simulink model "IMU_INS_Data"  (R2023b)
settings: Solver=VariableStepAuto  StartTime=0.0  StopTime=4  RelTol=1e-3
undefined symbols (not defined in the file): DiscIntNeverNeededParam, fractalcoef
libraries: simulink x3, sim3dautolib x2, mspsensorlib x1, sensorinslib x1, sim3dlib x1
settings Model: Creator=Hazem Abdelaziz  LastModifiedBy=Hazem Abdelaziz

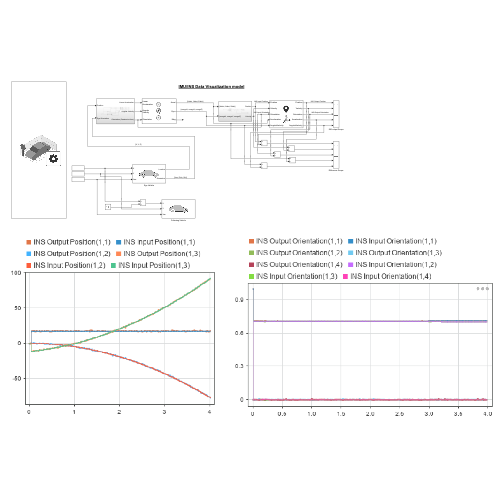
[thumbnail: Simulink's stored preview of the top-level diagram]
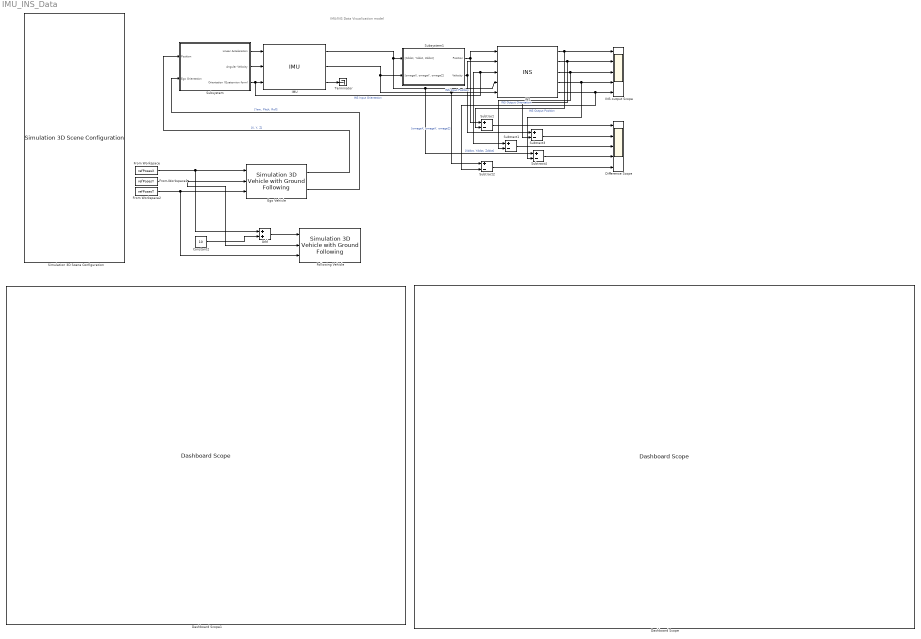
== system IMU_INS_Data ==
  note: IMU/INS Data Visualization model
  Add : Sum
  Constant2 : Constant  Value=10
  Dashboard Scope : DashboardScope  NormalizeYAxis=on
  Dashboard Scope1 : DashboardScope  NormalizeYAxis=on
  Difference Scope : Scope  NumInputPorts=5
  Ego Vehicle : sim3dautolib/Simulation 3D Vehicle with Ground Following  Priority=-1  PassVehMesh=Sedan  MeshPath=/MathWorksAutomotiveContent/Vehicles/Muscle/Meshes/SK_MuscleCar.SK_MuscleCar  TrackWidth=1.9  WheelBase=3  WheelRadius=0.35  VehColor=Black  InitialPos=[0, 0, 0]  InitialRot=[0, 0, 0]  ActorName=SimulinkVehicle1  SampleTime=-1  ActorType=SimulinkVehicle  ID=1  aMode=3  ActorTag=SimulinkVehicle1  CoordinateScheme=ISO  VehLightsControl=off  HeadlightColor=[ 1, 1, 1 ]  HighBeamIntensity=100000  LowBeamIntensity=60000  HighBeamConeAngle=70  LowBeamConeAngle=70  LeftHeadlightOrientation=[ 0, 0 ]  RightHeadlightOrientation=[ 0, 0 ]  BrakelightIntensity=500  ReverselightIntensity=500  SignallightIntensity=500  SignallightPeriod=1  SignalPulseWidth=50  TransformOutportEnabled=on
      settings: LibrarySourceBlock=drivingsim3d/Simulation 3D Vehicle with Ground Following
  Following Vehicle : sim3dautolib/Simulation 3D Vehicle with Ground Following  Priority=-1  PassVehMesh=Sedan  MeshPath=/MathWorksAutomotiveContent/Vehicles/Muscle/Meshes/SK_MuscleCar.SK_MuscleCar  TrackWidth=1.9  WheelBase=3  WheelRadius=0.35  VehColor=Red  InitialPos=[0, 0, 0]  InitialRot=[0, 0, 0]  ActorName=SimulinkVehicle2  SampleTime=-1  ActorType=SimulinkVehicle  ID=2  aMode=3  ActorTag=SimulinkVehicle2  CoordinateScheme=ISO  VehLightsControl=off  HeadlightColor=[ 1, 1, 1 ]  HighBeamIntensity=100000  LowBeamIntensity=60000  HighBeamConeAngle=70  LowBeamConeAngle=70  LeftHeadlightOrientation=[ 0, 0 ]  RightHeadlightOrientation=[ 0, 0 ]  BrakelightIntensity=500  ReverselightIntensity=500  SignallightIntensity=500  SignallightPeriod=1  SignalPulseWidth=50  TransformOutportEnabled=off
      settings: LibrarySourceBlock=drivingsim3d/Simulation 3D Vehicle with Ground Following
  From Workspace : FromWorkspace  VariableName=refPosesX  OutputAfterFinalValue=Holding final value
  From Workspace1 : FromWorkspace  VariableName=refPosesY  OutputAfterFinalValue=Holding final value
  From Workspace2 : FromWorkspace  VariableName=refPosesT  Interpolate=off  OutputAfterFinalValue=Holding final value
  IMU : mspsensorlib/IMU  DispRefFrame=ENU  TemperaturePort=off  Temperature=25  MagneticFieldPort=off  MagneticFieldNED=[ 27.5550, -2.4169, -16.0849 ]  MagneticFieldENU=[-2.4169, 27.5550, 16.0849]  SeedDouble=67  SimulateUsing=Interpreted execution  AccelParamsMeasurementRange=Inf  AccelParamsResolution=0  AccelParamsConstantBias=[ 0, 0, 9.81 ]  AccelParamsAxesMisalignment=[ 100, 0, 0; 0, 100, 0; 0, 0, 100 ]  AccelParamsNoiseDensity=[ 0, 0, 0 ]  AccelParamsBiasInstability=[ 0, 0, 0 ]  AccelParamsBiasInstabilityNumerator=fractalcoef().Numerator  AccelParamsBiasInstabilityDenominator=fractalcoef().Denominator  AccelParamsRandomWalk=[ 0, 0, 0 ]  AccelParamsNoiseType=double-sided  AccelParamsTemperatureBias=[ 0, 0, 0 ]  AccelParamsTemperatureScaleFactor=[ 0, 0, 0 ]  GyroParamsMeasurementRange=Inf  GyroParamsResolution=0  GyroParamsConstantBias=[ 0, 0, 0 ]  GyroParamsAxesMisalignment=[ 100, 0, 0; 0, 100, 0; 0, 0, 100 ]  GyroParamsAccelerationBias=[ 0, 0, 0 ]  GyroParamsNoiseDensity=[ 0, 0, 0 ]  GyroParamsBiasInstability=[ 0, 0, 0 ]  GyroParamsBiasInstabilityNumerator=fractalcoef().Numerator  GyroParamsBiasInstabilityDenominator=fractalcoef().Denominator  GyroParamsRandomWalk=[ 0, 0, 0 ]  GyroParamsNoiseType=double-sided  GyroParamsTemperatureBias=[ 0, 0, 0 ]  GyroParamsTemperatureScaleFactor=[ 0, 0, 0 ]  MagParamsMeasurementRange=Inf  MagParamsResolution=0  MagParamsConstantBias=[ 0, 0, 0 ]  MagParamsAxesMisalignment=[ 100, 0, 0; 0, 100, 0; 0, 0, 100 ]  MagParamsNoiseDensity=[ 0, 0, 0 ]  MagParamsBiasInstability=[ 0, 0, 0 ]  MagParamsBiasInstabilityNumerator=fractalcoef().Numerator  MagParamsBiasInstabilityDenominator=fractalcoef().Denominator  MagParamsRandomWalk=[ 0, 0, 0 ]  MagParamsNoiseType=double-sided  MagParamsTemperatureBias=[ 0, 0, 0 ]  MagParamsTemperatureScaleFactor=[ 0, 0, 0 ]
  INS : sensorinslib/INS  MountingLocation=[0 0 0]  RollAccuracy=0.05  PitchAccuracy=0.05  YawAccuracy=0.5  PositionAccuracy=0.5  VelocityAccuracy=0.05  UseAccelAndAngVel=on  AccelerationAccuracy=0.05  AngularVelocityAccuracy=0.05  TimeInput=off  PositionErrorFactor=[0 0 0]  SeedDouble=67  SimulateUsing=Code generation
      settings: LibrarySourceBlock=mspsensorlib/INS
  INS output Scope : Scope  NumInputPorts=5
  Simulation 3D Scene Configuration : sim3dlib/Simulation 3D Scene Configuration  Priority=0  ProjectFormat=Default Scenes  SceneDesc=US city block  ProjectName=C:\Program Files\MATLAB\R2023b\toolbox\shared\sim3d_projects\automotive_project_windows\UE\WindowsNoEditor\VehicleSimulation.exe  ScenePath=/Game/Maps/HwStrght  EnableOpenDRIVE=off  vehTagList={'Custom';'Scene Origin';'SimulinkVehicle1';'SimulinkVehicle2'}  vehTag=Scene Origin  FreeCameraInitialTranslation=[0, 0, 0]  FreeCameraDefaultInitialTranslation=[-6, 0, 2]  FreeCameraInitialRotation=[0, 0, 0]  FreeCameraDefaultInitialRotation=[0, -15, 0]  OpVisEn=off  Ts=1/60  EnableWindow=on  EnableRemoteAccess=off  EnableWeather=off  SunAltitude=40.0  SunAzimuth=90  clouds=10  wind=1  fog=0  rain=0  EnableGeospatial=off  OriginHeight=200  OriginLatitude=40.744652  OriginLongitude=-73.988864  MapStyle=Aerial  AdditionalAssetIDs=[]  UseAdvancedSunSky=off  SolarTime=11  TimeZone=-5  Day=21  Month=9  Year=2022  UseDaylightSavingTime=on  DSTStartDay=10  DSTStartMonth=3  DSTEndDay=3  DSTEndMonth=11  DSTSwitchHour=2  sensorTag=MainCamera1  sensorId=1  sensorName=MainCamera1  mountLoc=Origin  offsetFlag=off  tmountOffset=[0, 0, 0]  rmountOffset=[0, 0, 0]  HorizontalResolution=1280  VerticalResolution=720  HorizontalFOV=60  mountPoint=[0 0 0]  mountOrientation=[0 0 0]  aMode=3  ID=1  GeoTrigger=Inactive
      settings: LibrarySourceBlock=drivingsim3d/Simulation 3D Scene Configuration
  Subsystem : Subsystem
  Subsystem1 : Subsystem
  Subtract{,1..4} (5 alike) : Sum  Inputs=+-
  Terminator : Terminator
  wires:
  From Workspace/1 -> Add/1, Ego Vehicle/1
  From Workspace1/1 -> Following Vehicle/2, Ego Vehicle/2
  Add/1 -> Following Vehicle/1
  Constant2/1 -> Add/2
  From Workspace2/1 -> Following Vehicle/3, Ego Vehicle/3
  IMU/3 -> Terminator/1
  Ego Vehicle/1 -> Subsystem/1(Position)  "[X, Y, Z]"
  Ego Vehicle/2 -> Subsystem/2(Ego Orientation)  "[Yaw, Pitch, Roll]"
  Subsystem/1(Linear Acceleration) -> IMU/1
  Subsystem/2(Angular Velocity) -> IMU/2
  Subsystem/3(Orientation (Quaternion form)) -> INS/3, Subtract1/1, IMU/3  "INS Input Orientation"
  IMU/1 -> Subtract4/1, INS/4, Subsystem1/1("[Xddot, Yddot, Zddot]")  "[Xddot, Yddot, Zddot]"
  IMU/2 -> Subtract2/1, INS/5, Subsystem1/2("[omegaX, omegaY, omegaZ]")  "[omegaX, omegaY, omegaZ]"
  Subsystem1/1(Position) -> Subtract/1, INS/1  "INS Input Position"
  Subsystem1/2(Velocity) -> Subtract3/1, INS/2
  INS/1 -> Subtract/2, INS output Scope/1  "INS Output Position"
  INS/2 -> Subtract3/2, INS output Scope/2
  INS/3 -> Subtract1/2, INS output Scope/3  "INS Output Orientation"
  INS/4 -> INS output Scope/4, Subtract4/2
  INS/5 -> Subtract2/2, INS output Scope/5
  Subtract2/1 -> Difference Scope/5
  Subtract/1 -> Difference Scope/1
  Subtract1/1 -> Difference Scope/3
  Subtract4/1 -> Difference Scope/4
  Subtract3/1 -> Difference Scope/2

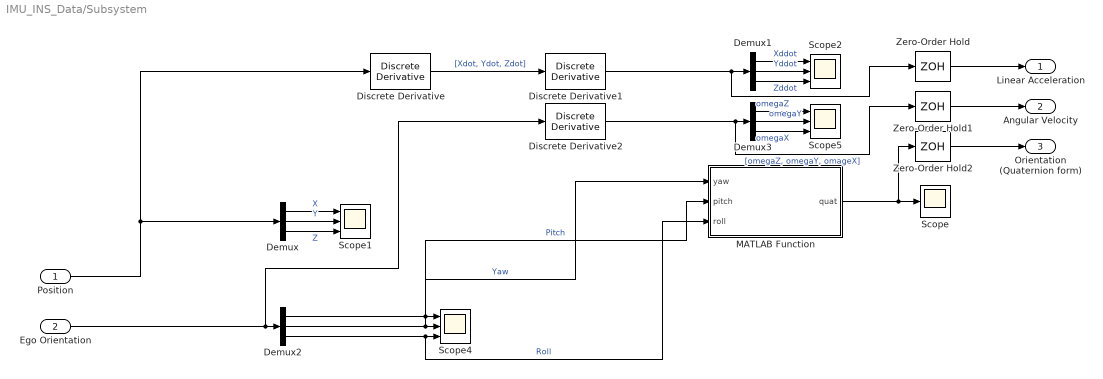
== system IMU_INS_Data/Subsystem ==
  Position : Inport
  Ego Orientation : Inport  Port=2
  Demux{,1..3} (4 alike) : Demux  Outputs=3
  Discrete Derivative : simulink/Discrete/Discrete Derivative  gainval=1.0  ICPrevScaledInput=0.0  OutMin=[]  OutMax=[]  OutDataType=fixdt(1, 16)  OutScaling=2^-10  DoSatur=off
  Discrete Derivative1 : simulink/Discrete/Discrete Derivative  gainval=1.0  ICPrevScaledInput=0.0  OutMin=[]  OutMax=[]  OutDataType=fixdt(1, 16)  OutScaling=2^-10  DoSatur=off
  Discrete Derivative2 : simulink/Discrete/Discrete Derivative  gainval=1.0  ICPrevScaledInput=0.0  OutMin=[]  OutMax=[]  OutDataType=fixdt(1, 16)  OutScaling=2^-10  DoSatur=off
  MATLAB Function : MATLAB Function  TreatAsAtomicUnit=on
  Scope : Scope
  Scope{1..2,4..5} (4 alike) : Scope  NumInputPorts=3
  Zero-Order Hold : ZeroOrderHold  SampleTime=-1
  Zero-Order Hold1 : ZeroOrderHold  SampleTime=-1
  Zero-Order Hold2 : ZeroOrderHold  SampleTime=-1
  Linear Acceleration : Outport
  Angular Velocity : Outport  Port=2
  Orientation (Quaternion form) : Outport  Port=3
  wires:
  Demux1/1 -> Scope2/1  "Xddot"
  Discrete Derivative/1 -> Discrete Derivative1/1  "[Xdot, Ydot, Zdot]"
  Zero-Order Hold2/1 -> Orientation (Quaternion form)/1
  Demux2/1 -> Scope4/1, MATLAB Function/1(yaw)  "Yaw"
  Discrete Derivative2/1 -> Zero-Order Hold1/1, Demux3/1  "[omegaZ, omegaY, omageX]"
  Ego Orientation/1 -> Discrete Derivative2/1, Demux2/1
  Demux2/3 -> MATLAB Function/3(roll), Scope4/3  "Roll"
  Demux1/3 -> Scope2/3  "Zddot"
  Demux2/2 -> MATLAB Function/2(pitch), Scope4/2  "Pitch"
  Discrete Derivative1/1 -> Zero-Order Hold/1, Demux1/1
  Demux3/3 -> Scope5/3  "omegaX"
  Demux/2 -> Scope1/2  "Y"
  Zero-Order Hold/1 -> Linear Acceleration/1
  Demux3/1 -> Scope5/1  "omegaZ"
  MATLAB Function/1(quat) -> Zero-Order Hold2/1, Scope/1
  Demux/1 -> Scope1/1  "X"
  Demux1/2 -> Scope2/2  "Yddot"
  Position/1 -> Discrete Derivative/1, Demux/1
  Demux3/2 -> Scope5/2  "omegaY"
  Demux/3 -> Scope1/3  "Z"
  Zero-Order Hold1/1 -> Angular Velocity/1

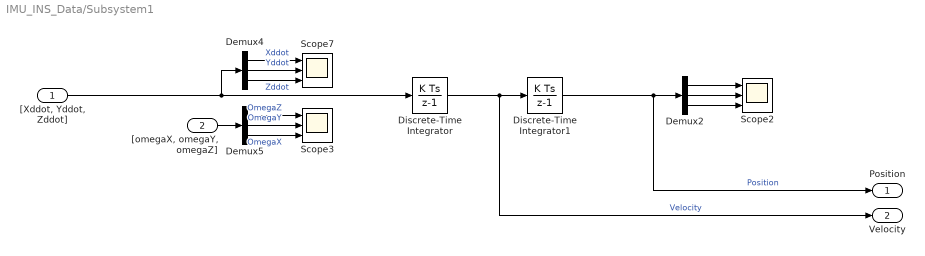
== system IMU_INS_Data/Subsystem1 ==
  "[Xddot, Yddot, Zddot]" : Inport
  "[omegaX, omegaY, omegaZ]" : Inport  Port=2
  Demux2 : Demux  Outputs=3
  Demux4 : Demux  Outputs=3
  Demux5 : Demux  Outputs=3
  Discrete-Time Integrator : DiscreteIntegrator  SampleTime=-1  ICPrevOutput=DiscIntNeverNeededParam  ICPrevScaledInput=DiscIntNeverNeededParam
  Discrete-Time Integrator1 : DiscreteIntegrator  SampleTime=-1  ICPrevOutput=DiscIntNeverNeededParam  ICPrevScaledInput=DiscIntNeverNeededParam
  Scope2 : Scope  NumInputPorts=3
  Scope3 : Scope  NumInputPorts=3
  Scope7 : Scope  NumInputPorts=3
  Position : Outport
  Velocity : Outport  Port=2
  wires:
  Demux5/1 -> Scope3/1  "OmegaZ"
  Demux4/2 -> Scope7/2  "Yddot"
  Discrete-Time Integrator1/1 -> Position/1, Demux2/1  "Position"
  Discrete-Time Integrator/1 -> Velocity/1, Discrete-Time Integrator1/1  "Velocity"
  Demux2/3 -> Scope2/3
  Demux4/3 -> Scope7/3  "Zddot"
  Demux5/3 -> Scope3/3  "OmegaX"
  Demux4/1 -> Scope7/1  "Xddot"
  Demux5/2 -> Scope3/2  "OmegaY"
  "[Xddot, Yddot, Zddot]"/1 -> Demux4/1, Discrete-Time Integrator/1
  Demux2/1 -> Scope2/1
  Demux2/2 -> Scope2/2
  "[omegaX, omegaY, omegaZ]"/1 -> Demux5/1

== matlab function IMU_INS_Data/Subsystem/MATLAB Function ==
  data: yaw input; quat output; pitch input; roll input
function quat = euler_to_quaternion(yaw, pitch, roll)
    %Converting Euler angles to quaternion


    % Compute quaternion components
    cy = cos(yaw * 0.5);
    sy = sin(yaw * 0.5);
    cp = cos(pitch * 0.5);
    sp = sin(pitch * 0.5);
    cr = cos(roll * 0.5);
    sr = sin(roll * 0.5);

    % Quaternion elements
    qw = cy * cp * cr + sy * sp * sr;
    qx = cy * cp * sr - sy * sp * cr;
    qy = sy * cp * sr + cy * sp * cr;
    qz = sy * cp * cr - cy * sp * sr;

    % Output quaternion
    quat = [qw, qx, qy, qz];
